simulink model "gnss_arch"  (R2021a)
settings: Solver=FixedStepDiscrete  StartTime=0.0  StopTime=10.0  RelTol=1e-3
undefined symbols (not defined in the file): BASE, CONFIG, DATA, FILE, NAV, OBS, RAW, ROVER
settings Model: Creator=Marcos  LastModifiedBy=Marcos

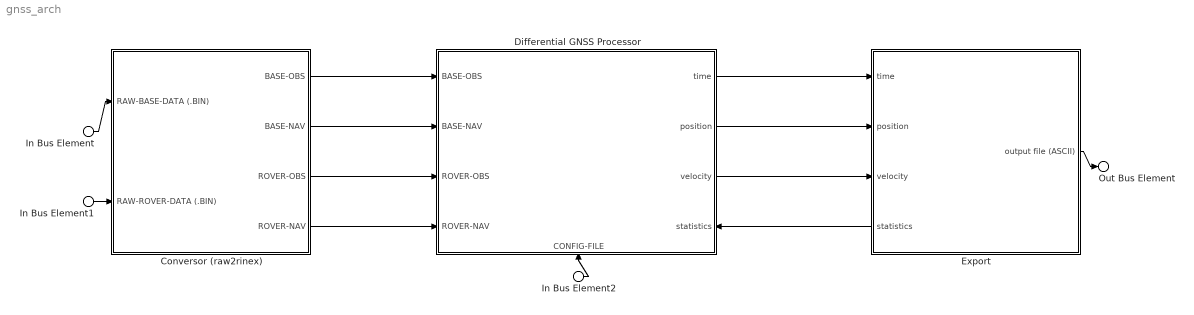
== system gnss_arch ==
  In Bus Element : Inport  PortName=RAW-BASE-DATA (.BIN)
  In Bus Element2 : Inport  Port=2  PortName=CONFIG-FILE
  In Bus Element1 : Inport  Port=3  PortName=RAW-ROVER-DATA (.BIN)
  Conversor (raw2rinex) : Subsystem
      settings: PortSchema="{\"entries\":[{\"content\":{\"headerSize\":26,\"margin\":15,\"minimumSpacing\":25,\"sides\":[{\"content\":{\"connectorIds\":[\"In1\",\"In2\"]},\"type\":\"ConnectorPlacement.EquallySpacedRectSide\",\"uuid\":\"3b3b2daf-559c-4471-8efc-02c8e3f1b512\"},{\"content\":{\"connectorIds\":[\"Out1\",\"Out2\",\"Out3\",\"Out4\"],\"side\":\"RIGHT\"},\"type\":\"ConnectorPlacement.EquallySpacedRectSide\",\"uuid\":\"f23ce325-f635-4381-8a74-1aafa4556df0\"},{\"content\":{\"connectorIds\":[],\"side\":\"TOP\"},\"type\":\"ConnectorPlacement.EquallySpacedRectSide\",\"uuid\":\"eecd7f47-80e4-47d6-b093-9e794683967f\"}]},\"type\":\"ConnectorPlacement.EquallySpacedConnector\",\"uuid\":\"6f862817-9114-4679-9a94-508ae26eea16\"}],\"packageUris\":[\"http://schema.mathworks.com/mf0/Connector/R2020b\"],\"version\":\"1.0\"}"
  Differential GNSS Processor : Subsystem
      settings: PortSchema="{\"entries\":[{\"content\":{\"headerSize\":26,\"margin\":15,\"minimumSpacing\":25,\"sides\":[{\"content\":{\"connectorIds\":[\"In3\",\"In4\",\"In5\",\"In6\"]},\"type\":\"ConnectorPlacement.EquallySpacedRectSide\",\"uuid\":\"3b3b2daf-559c-4471-8efc-02c8e3f1b512\"},{\"content\":{\"connectorIds\":[\"Out1\",\"Out2\",\"Out3\",\"In2\"],\"side\":\"RIGHT\"},\"type\":\"ConnectorPlacement.EquallySpacedRectSide\",\"uuid\":\"f23ce325-f635-4381-8a74-1aafa4556df0\"},{\"content\":{\"connectorIds\":[],\"side\":\"TOP\"},\"type\":\"ConnectorPlacement.EquallySpacedRectSide\",\"uuid\":\"eecd7f47-80e4-47d6-b093-9e794683967f\"},{\"content\":{\"connectorIds\":[\"In1\"],\"side\":\"BOTTOM\"},\"type\":\"ConnectorPlacement.EquallySpacedRectSide\",\"uuid\":\"dadb23e3-3510-4639-8845-4c2e23d1ffa2\"}]},\"type\":\"ConnectorPlacement.EquallySpacedConnector\",\"uuid\":\"6f862817-9114-4679-9a94-508ae26eea16\"}],\"packageUris\":[\"http://schema.mathworks.com/mf0/Connector/R2020b\"],\"version\":\"1.0\"}"
  Export : Subsystem
      settings: PortSchema="{\"entries\":[{\"content\":{\"headerSize\":26,\"margin\":15,\"minimumSpacing\":25,\"sides\":[{\"content\":{\"connectorIds\":[\"In1\",\"In2\",\"In3\",\"Out2\"]},\"type\":\"ConnectorPlacement.EquallySpacedRectSide\",\"uuid\":\"3b3b2daf-559c-4471-8efc-02c8e3f1b512\"},{\"content\":{\"connectorIds\":[\"Out1\"],\"side\":\"RIGHT\"},\"type\":\"ConnectorPlacement.EquallySpacedRectSide\",\"uuid\":\"f23ce325-f635-4381-8a74-1aafa4556df0\"},{\"content\":{\"connectorIds\":[],\"side\":\"TOP\"},\"type\":\"ConnectorPlacement.EquallySpacedRectSide\",\"uuid\":\"eecd7f47-80e4-47d6-b093-9e794683967f\"}]},\"type\":\"ConnectorPlacement.EquallySpacedConnector\",\"uuid\":\"6f862817-9114-4679-9a94-508ae26eea16\"}],\"packageUris\":[\"http://schema.mathworks.com/mf0/Connector/R2020b\"],\"version\":\"1.0\"}"
  Out Bus Element : Outport  PortName=output file (ASCII)
  wires:
  In Bus Element/1 -> Conversor (raw2rinex)/1(RAW-BASE-DATA (.BIN))
  In Bus Element1/1 -> Conversor (raw2rinex)/2(RAW-ROVER-DATA (.BIN))
  Conversor (raw2rinex)/3(ROVER-OBS) -> Differential GNSS Processor/5(ROVER-OBS)
  Conversor (raw2rinex)/4(ROVER-NAV) -> Differential GNSS Processor/6(ROVER-NAV)
  Conversor (raw2rinex)/1(BASE-OBS) -> Differential GNSS Processor/3(BASE-OBS)
  Conversor (raw2rinex)/2(BASE-NAV) -> Differential GNSS Processor/4(BASE-NAV)
  Differential GNSS Processor/1(time) -> Export/1(time)
  Differential GNSS Processor/2(position) -> Export/2(position)
  Differential GNSS Processor/3(velocity) -> Export/3(velocity)
  Export/2(statistics) -> Differential GNSS Processor/2(statistics)
  Export/1(output file (ASCII)) -> Out Bus Element/1
  In Bus Element2/1 -> Differential GNSS Processor/1(CONFIG-FILE)

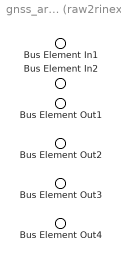
== system gnss_arch/Conversor (raw2rinex) ==
  Bus Element In1 : Inport  PortName=RAW-BASE-DATA (.BIN)
  Bus Element In2 : Inport  Port=2  PortName=RAW-ROVER-DATA (.BIN)
  Bus Element Out1 : Outport  PortName=BASE-OBS
  Bus Element Out2 : Outport  Port=2  PortName=BASE-NAV
  Bus Element Out3 : Outport  Port=3  PortName=ROVER-OBS
  Bus Element Out4 : Outport  Port=4  PortName=ROVER-NAV

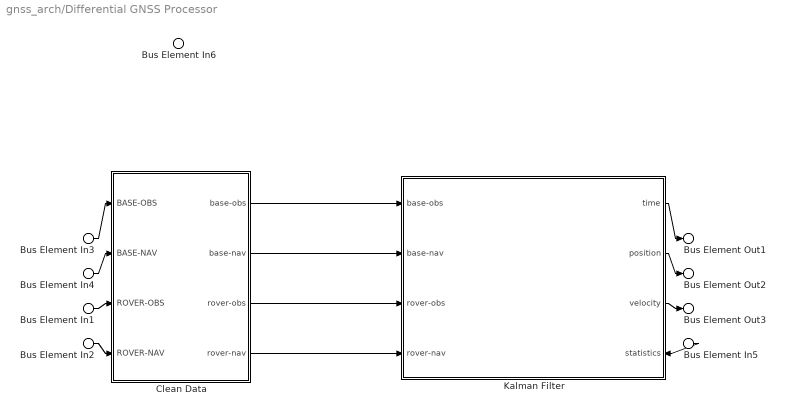
== system gnss_arch/Differential GNSS Processor ==
  Bus Element In6 : Inport  PortName=CONFIG-FILE
  Bus Element In5 : Inport  Port=2  PortName=statistics
  Bus Element In3 : Inport  Port=3  PortName=BASE-OBS
  Bus Element In4 : Inport  Port=4  PortName=BASE-NAV
  Bus Element In1 : Inport  Port=5  PortName=ROVER-OBS
  Bus Element In2 : Inport  Port=6  PortName=ROVER-NAV
  Clean Data : Subsystem
      settings: PortSchema="{\"entries\":[{\"content\":{\"headerSize\":26,\"margin\":15,\"minimumSpacing\":25,\"sides\":[{\"content\":{\"connectorIds\":[\"In1\",\"In2\",\"In3\",\"In4\"]},\"type\":\"ConnectorPlacement.EquallySpacedRectSide\",\"uuid\":\"3b3b2daf-559c-4471-8efc-02c8e3f1b512\"},{\"content\":{\"connectorIds\":[\"Out1\",\"Out2\",\"Out3\",\"Out4\"],\"side\":\"RIGHT\"},\"type\":\"ConnectorPlacement.EquallySpacedRectSide\",\"uuid\":\"f23ce325-f635-4381-8a74-1aafa4556df0\"},{\"content\":{\"connectorIds\":[],\"side\":\"TOP\"},\"type\":\"ConnectorPlacement.EquallySpacedRectSide\",\"uuid\":\"eecd7f47-80e4-47d6-b093-9e794683967f\"}]},\"type\":\"ConnectorPlacement.EquallySpacedConnector\",\"uuid\":\"6f862817-9114-4679-9a94-508ae26eea16\"}],\"packageUris\":[\"http://schema.mathworks.com/mf0/Connector/R2020b\"],\"version\":\"1.0\"}"
  Kalman Filter : Subsystem
      settings: PortSchema="{\"entries\":[{\"content\":{\"headerSize\":26,\"margin\":15,\"minimumSpacing\":25,\"sides\":[{\"content\":{\"connectorIds\":[\"In1\",\"In2\",\"In3\",\"In4\"]},\"type\":\"ConnectorPlacement.EquallySpacedRectSide\",\"uuid\":\"3b3b2daf-559c-4471-8efc-02c8e3f1b512\"},{\"content\":{\"connectorIds\":[\"Out1\",\"Out2\",\"Out3\",\"In5\"],\"side\":\"RIGHT\"},\"type\":\"ConnectorPlacement.EquallySpacedRectSide\",\"uuid\":\"f23ce325-f635-4381-8a74-1aafa4556df0\"},{\"content\":{\"connectorIds\":[],\"side\":\"TOP\"},\"type\":\"ConnectorPlacement.EquallySpacedRectSide\",\"uuid\":\"eecd7f47-80e4-47d6-b093-9e794683967f\"}]},\"type\":\"ConnectorPlacement.EquallySpacedConnector\",\"uuid\":\"6f862817-9114-4679-9a94-508ae26eea16\"}],\"packageUris\":[\"http://schema.mathworks.com/mf0/Connector/R2020b\"],\"version\":\"1.0\"}"
  Bus Element Out1 : Outport  PortName=time
  Bus Element Out2 : Outport  Port=2  PortName=position
  Bus Element Out3 : Outport  Port=3  PortName=velocity
  wires:
  Bus Element In3/1 -> Clean Data/1(BASE-OBS)
  Bus Element In4/1 -> Clean Data/2(BASE-NAV)
  Bus Element In1/1 -> Clean Data/3(ROVER-OBS)
  Bus Element In2/1 -> Clean Data/4(ROVER-NAV)
  Kalman Filter/1(time) -> Bus Element Out1/1
  Kalman Filter/2(position) -> Bus Element Out2/1
  Kalman Filter/3(velocity) -> Bus Element Out3/1
  Bus Element In5/1 -> Kalman Filter/5(statistics)
  Clean Data/1(base-obs) -> Kalman Filter/1(base-obs)
  Clean Data/2(base-nav) -> Kalman Filter/2(base-nav)
  Clean Data/3(rover-obs) -> Kalman Filter/3(rover-obs)
  Clean Data/4(rover-nav) -> Kalman Filter/4(rover-nav)

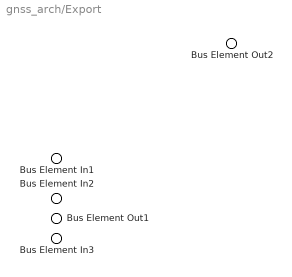
== system gnss_arch/Export ==
  Bus Element In1 : Inport  PortName=time
  Bus Element In2 : Inport  Port=2  PortName=position
  Bus Element In3 : Inport  Port=3  PortName=velocity
  Bus Element Out2 : Outport  PortName=output file (ASCII)
  Bus Element Out1 : Outport  Port=2  PortName=statistics

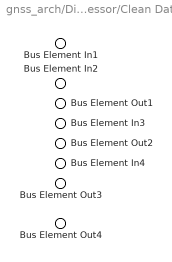
== system gnss_arch/Differential GNSS Processor/Clean Data ==
  Bus Element In1 : Inport  PortName=BASE-OBS
  Bus Element In2 : Inport  Port=2  PortName=BASE-NAV
  Bus Element In3 : Inport  Port=3  PortName=ROVER-OBS
  Bus Element In4 : Inport  Port=4  PortName=ROVER-NAV
  Bus Element Out1 : Outport  PortName=base-obs
  Bus Element Out2 : Outport  Port=2  PortName=base-nav
  Bus Element Out3 : Outport  Port=3  PortName=rover-obs
  Bus Element Out4 : Outport  Port=4  PortName=rover-nav

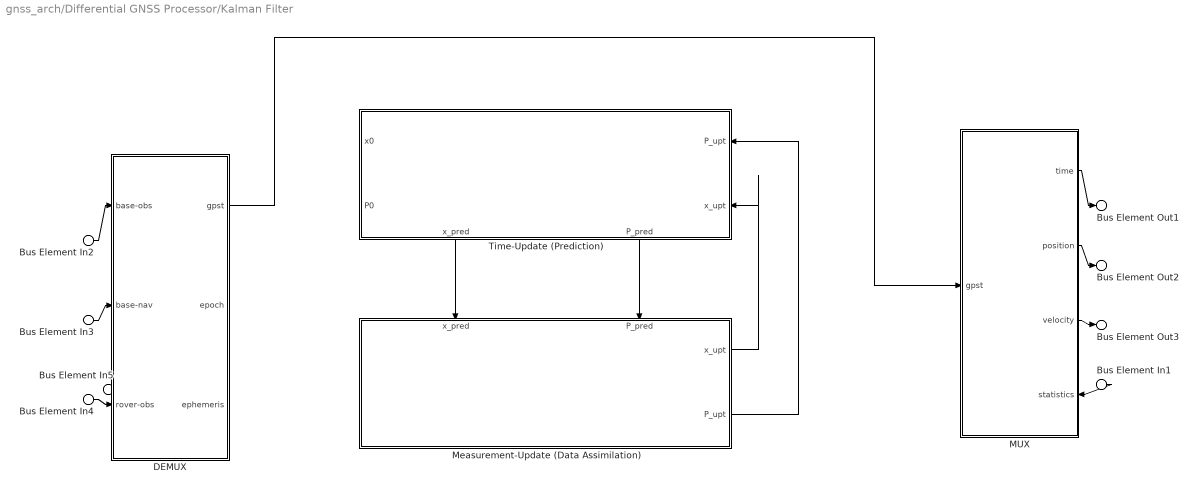
== system gnss_arch/Differential GNSS Processor/Kalman Filter ==
  Bus Element In2 : Inport  PortName=base-obs
  Bus Element In3 : Inport  Port=2  PortName=base-nav
  Bus Element In4 : Inport  Port=3  PortName=rover-obs
  Bus Element In5 : Inport  Port=4  PortName=rover-nav
  Bus Element In1 : Inport  Port=5  PortName=statistics
  DEMUX : Subsystem
      settings: PortSchema="{\"entries\":[{\"content\":{\"headerSize\":26,\"margin\":15,\"minimumSpacing\":25,\"sides\":[{\"content\":{\"connectorIds\":[\"In1\",\"In2\",\"In3\"]},\"type\":\"ConnectorPlacement.EquallySpacedRectSide\",\"uuid\":\"3b3b2daf-559c-4471-8efc-02c8e3f1b512\"},{\"content\":{\"connectorIds\":[\"Out1\",\"Out2\",\"Out3\"],\"side\":\"RIGHT\"},\"type\":\"ConnectorPlacement.EquallySpacedRectSide\",\"uuid\":\"f23ce325-f635-4381-8a74-1aafa4556df0\"},{\"content\":{\"connectorIds\":[],\"side\":\"TOP\"},\"type\":\"ConnectorPlacement.EquallySpacedRectSide\",\"uuid\":\"eecd7f47-80e4-47d6-b093-9e794683967f\"}]},\"type\":\"ConnectorPlacement.EquallySpacedConnector\",\"uuid\":\"6f862817-9114-4679-9a94-508ae26eea16\"}],\"packageUris\":[\"http://schema.mathworks.com/mf0/Connector/R2020b\"],\"version\":\"1.0\"}"
  MUX : Subsystem
      settings: PortSchema="{\"entries\":[{\"content\":{\"headerSize\":26,\"margin\":15,\"minimumSpacing\":25,\"sides\":[{\"content\":{\"connectorIds\":[\"In1\"]},\"type\":\"ConnectorPlacement.EquallySpacedRectSide\",\"uuid\":\"3b3b2daf-559c-4471-8efc-02c8e3f1b512\"},{\"content\":{\"connectorIds\":[\"Out1\",\"Out2\",\"Out3\",\"In2\"],\"side\":\"RIGHT\"},\"type\":\"ConnectorPlacement.EquallySpacedRectSide\",\"uuid\":\"f23ce325-f635-4381-8a74-1aafa4556df0\"},{\"content\":{\"connectorIds\":[],\"side\":\"TOP\"},\"type\":\"ConnectorPlacement.EquallySpacedRectSide\",\"uuid\":\"eecd7f47-80e4-47d6-b093-9e794683967f\"}]},\"type\":\"ConnectorPlacement.EquallySpacedConnector\",\"uuid\":\"6f862817-9114-4679-9a94-508ae26eea16\"}],\"packageUris\":[\"http://schema.mathworks.com/mf0/Connector/R2020b\"],\"version\":\"1.0\"}"
  Measurement-Update (Data Assimilation) : Subsystem
      settings: PortSchema="{\"entries\":[{\"content\":{\"headerSize\":26,\"margin\":15,\"minimumSpacing\":25,\"sides\":[{\"content\":{\"connectorIds\":[]},\"type\":\"ConnectorPlacement.EquallySpacedRectSide\",\"uuid\":\"3b3b2daf-559c-4471-8efc-02c8e3f1b512\"},{\"content\":{\"connectorIds\":[\"Out1\",\"Out2\"],\"side\":\"RIGHT\"},\"type\":\"ConnectorPlacement.EquallySpacedRectSide\",\"uuid\":\"f23ce325-f635-4381-8a74-1aafa4556df0\"},{\"content\":{\"connectorIds\":[\"In1\",\"In2\"],\"side\":\"TOP\"},\"type\":\"ConnectorPlacement.EquallySpacedRectSide\",\"uuid\":\"eecd7f47-80e4-47d6-b093-9e794683967f\"}]},\"type\":\"ConnectorPlacement.EquallySpacedConnector\",\"uuid\":\"6f862817-9114-4679-9a94-508ae26eea16\"}],\"packageUris\":[\"http://schema.mathworks.com/mf0/Connector/R2020b\"],\"version\":\"1.0\"}"
  Time-Update (Prediction) : Subsystem
      settings: PortSchema="{\"entries\":[{\"content\":{\"headerSize\":26,\"margin\":15,\"minimumSpacing\":25,\"sides\":[{\"content\":{\"connectorIds\":[\"In2\",\"In3\"]},\"type\":\"ConnectorPlacement.EquallySpacedRectSide\",\"uuid\":\"3b3b2daf-559c-4471-8efc-02c8e3f1b512\"},{\"content\":{\"connectorIds\":[\"In1\",\"In4\"],\"side\":\"RIGHT\"},\"type\":\"ConnectorPlacement.EquallySpacedRectSide\",\"uuid\":\"f23ce325-f635-4381-8a74-1aafa4556df0\"},{\"content\":{\"connectorIds\":[],\"side\":\"TOP\"},\"type\":\"ConnectorPlacement.EquallySpacedRectSide\",\"uuid\":\"eecd7f47-80e4-47d6-b093-9e794683967f\"},{\"content\":{\"connectorIds\":[\"Out1\",\"Out2\"],\"side\":\"BOTTOM\"},\"type\":\"ConnectorPlacement.EquallySpacedRectSide\",\"uuid\":\"7b683590-0e3b-4c29-b883-44f730959ce3\"}]},\"type\":\"ConnectorPlacement.EquallySpacedConnector\",\"uuid\":\"6f862817-9114-4679-9a94-508ae26eea16\"}],\"packageUris\":[\"http://schema.mathworks.com/mf0/Connector/R2020b\"],\"version\":\"1.0\"}"
  Bus Element Out1 : Outport  PortName=time
  Bus Element Out2 : Outport  Port=2  PortName=position
  Bus Element Out3 : Outport  Port=3  PortName=velocity
  wires:
  Bus Element In2/1 -> DEMUX/1(base-obs)
  Bus Element In3/1 -> DEMUX/2(base-nav)
  Bus Element In4/1 -> DEMUX/3(rover-obs)
  Time-Update (Prediction)/1(x_pred) -> Measurement-Update (Data Assimilation)/1(x_pred)
  Time-Update (Prediction)/2(P_pred) -> Measurement-Update (Data Assimilation)/2(P_pred)
  Measurement-Update (Data Assimilation)/1(x_upt) -> Time-Update (Prediction)/4(x_upt)
  Measurement-Update (Data Assimilation)/2(P_upt) -> Time-Update (Prediction)/1(P_upt)
  MUX/1(time) -> Bus Element Out1/1
  MUX/2(position) -> Bus Element Out2/1
  MUX/3(velocity) -> Bus Element Out3/1
  Bus Element In1/1 -> MUX/2(statistics)
  DEMUX/1(gpst) -> MUX/1(gpst)

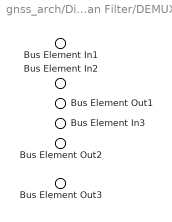
== system gnss_arch/Differential GNSS Processor/Kalman Filter/DEMUX ==
  Bus Element In1 : Inport  PortName=base-obs
  Bus Element In2 : Inport  Port=2  PortName=base-nav
  Bus Element In3 : Inport  Port=3  PortName=rover-obs
  Bus Element Out1 : Outport  PortName=gpst
  Bus Element Out2 : Outport  Port=2  PortName=epoch
  Bus Element Out3 : Outport  Port=3  PortName=ephemeris

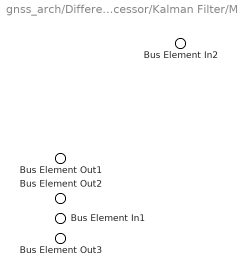
== system gnss_arch/Differential GNSS Processor/Kalman Filter/MUX ==
  Bus Element In2 : Inport  PortName=gpst
  Bus Element In1 : Inport  Port=2  PortName=statistics
  Bus Element Out1 : Outport  PortName=time
  Bus Element Out2 : Outport  Port=2  PortName=position
  Bus Element Out3 : Outport  Port=3  PortName=velocity

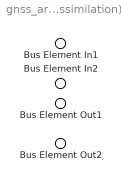
== system gnss_arch/Differential GNSS Processor/Kalman Filter/Measurement-Update (Data Assimilation) ==
  Bus Element In1 : Inport  PortName=x_pred
  Bus Element In2 : Inport  Port=2  PortName=P_pred
  Bus Element Out1 : Outport  PortName=x_upt
  Bus Element Out2 : Outport  Port=2  PortName=P_upt

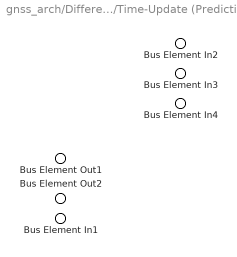
== system gnss_arch/Differential GNSS Processor/Kalman Filter/Time-Update (Prediction) ==
  Bus Element In4 : Inport  PortName=P_upt
  Bus Element In2 : Inport  Port=2  PortName=x0
  Bus Element In3 : Inport  Port=3  PortName=P0
  Bus Element In1 : Inport  Port=4  PortName=x_upt
  Bus Element Out1 : Outport  PortName=x_pred
  Bus Element Out2 : Outport  Port=2  PortName=P_pred
